simulink model "vloop_test2"  (Simulink 7.5)
settings: Solver=ode15s  StartTime=0.0  StopTime=1.0  RelTol=1e-3
InitFcn:
  | G = 107.815;
libraries: control x1
settings Model: Creator=pic  LastModifiedBy=corkep
settings DebuggingCC: StrictBusMsg=Warning
settings SFSimCC: SimCustomInitializer=|
  | if ~exist(tau_d)
  |    tau_d = 0
  | end

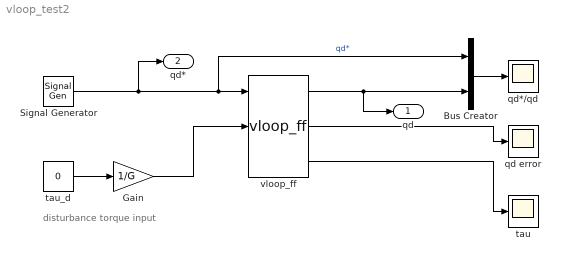
== system vloop_test2 ==
  note: disturbance torque input
  Bus Creator : BusCreator  Inputs=2
  Gain : Gain  Gain=1/G  ParameterDataType=fixdt(1, 16)  ParameterScaling=2^0  OutDataType=fixdt(1, 16)  OutScaling=2^0
  Signal Generator : SignalGenerator  WaveForm=sawtooth  Frequency=2
  qd error : Scope
      settings: TimeRange=1  YMin=0  YMax=0.7  SaveName=ScopeData2
  qd*/qd : Scope
      settings: TimeRange=1  YMin=0  YMax=90
  tau : Scope
      settings: TimeRange=1  YMin=-0.1  YMax=0.175
  tau_d : Constant  Value=0  OutDataType=fixdt(1, 16)  OutScaling=2^0
  vloop_ff : control/vloop_ff  SystemSampleTime=-1  J=372e-6  B=817e-6  Km=0.228  tau_max=0.9  Kv=1  Ki=0  T=0.001
  qd : Outport  OutDataType=fixdt(1, 16)  OutScaling=2^0
  qd* : Outport  Port=2  OutDataType=fixdt(1, 16)  OutScaling=2^0
  wires:
  Signal Generator/1 -> qd*/1, Bus Creator/1, vloop_ff/1  "qd*"
  Bus Creator/1 -> qd*/qd/1
  tau_d/1 -> Gain/1
  vloop_ff/1 -> Bus Creator/2, qd/1
  vloop_ff/2 -> qd error/1
  vloop_ff/3 -> tau/1
  Gain/1 -> vloop_ff/2
